simulink model "vehicleXYsim"  (R2018b)
settings: Solver=FixedStepAuto  StartTime=0.0  StopTime=end_time  FixedStep=0.1  RelTol=1e-3
libraries: simulink x2, vehdynlibviscommon x1
settings Model: Creator=mk  LastModifiedBy=mk

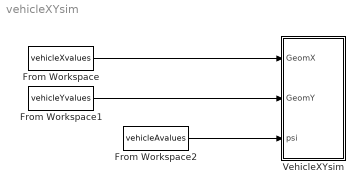
== system vehicleXYsim ==
  From Workspace : FromWorkspace  VariableName=vehicleXvalues  SampleTime=0
  From Workspace1 : FromWorkspace  VariableName=vehicleYvalues  SampleTime=0
  From Workspace2 : FromWorkspace  VariableName=vehicleAvalues  SampleTime=0
  VehicleXYsim : Subsystem
  wires:
  From Workspace/1 -> VehicleXYsim/1(GeomX)
  From Workspace1/1 -> VehicleXYsim/2(GeomY)
  From Workspace2/1 -> VehicleXYsim/3(psi)

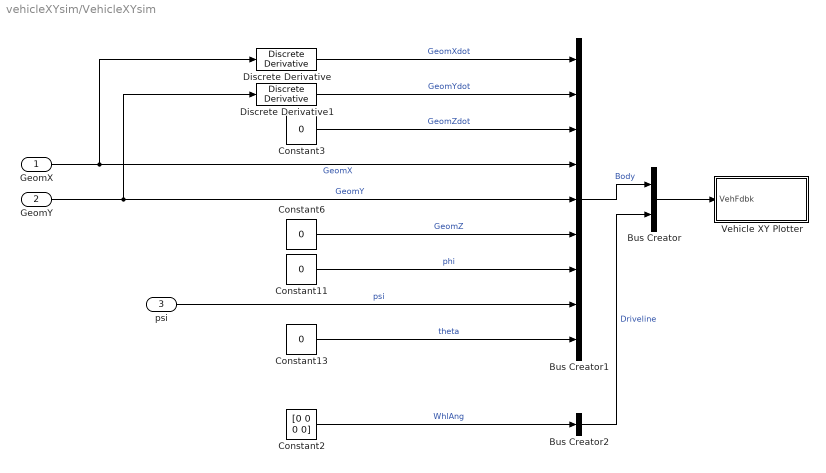
== system vehicleXYsim/VehicleXYsim ==
  GeomX : Inport
  GeomY : Inport  Port=2
  psi : Inport  Port=3
  Bus Creator : BusCreator  Inputs=2
  Bus Creator1 : BusCreator  Inputs=9
  Bus Creator2 : BusCreator  Inputs=1
  Constant{3,6,11,13} (4 alike) : Constant  Value=0
  Constant2 : Constant  Value=[0 0 0 0]
  Discrete Derivative : simulink/Discrete/Discrete Derivative  gainval=1.0  ICPrevScaledInput=0.0  OutMin=[]  OutMax=[]  OutDataType=fixdt(1, 16)  OutScaling=2^-10  DoSatur=off
  Discrete Derivative1 : simulink/Discrete/Discrete Derivative  gainval=1.0  ICPrevScaledInput=0.0  OutMin=[]  OutMax=[]  OutDataType=fixdt(1, 16)  OutScaling=2^-10  DoSatur=off
  Vehicle XY Plotter : Subsystem  mask(Vehicle XY Plotter){a=0.5, b=0.5, w=0.75, figBorder=10, bufferSize=1024, pltDT=.1}
      mask prompts: a "Distance to front axle from CG, a [m]:"; b "Distance to rear axle from CG, b [m]:"; w "Track width, w [m]:"; figBorder "Distance to figure borders, figBorder [m]:"; bufferSize "Path buffer sampe size, bufferSize []:"; pltDT "Plot update rate, pltDT [s]:"
      mask help: This block will display a MATLAB figure which indicates the vehicle path, current position and heading velocity.
      mask TypeOptions a: Vehicle XY Plotter/a
      mask TypeOptions b: Vehicle XY Plotter/b
      mask TypeOptions w: Vehicle XY Plotter/w
      mask TypeOptions figBorder: Vehicle XY Plotter/figBorder
      mask TypeOptions bufferSize: Vehicle XY Plotter/bufferSize
  wires:
  Discrete Derivative/1 -> Bus Creator1/1  "GeomXdot"
  GeomY/1 -> Discrete Derivative1/1, Bus Creator1/5  "GeomY"
  Constant3/1 -> Bus Creator1/3  "GeomZdot"
  Constant6/1 -> Bus Creator1/6  "GeomZ"
  GeomX/1 -> Discrete Derivative/1, Bus Creator1/4  "GeomX"
  Constant11/1 -> Bus Creator1/7  "phi"
  Constant2/1 -> Bus Creator2/1  "WhlAng"
  Constant13/1 -> Bus Creator1/9  "theta"
  Discrete Derivative1/1 -> Bus Creator1/2  "GeomYdot"
  Bus Creator2/1 -> Bus Creator/2  "Driveline"
  Bus Creator/1 -> Vehicle XY Plotter/1(VehFdbk)
  psi/1 -> Bus Creator1/8  "psi"
  Bus Creator1/1 -> Bus Creator/1  "Body"

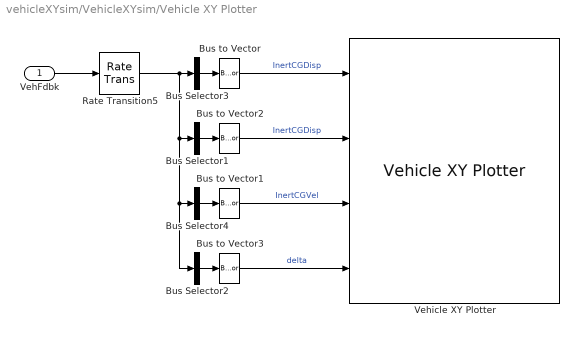
== system vehicleXYsim/VehicleXYsim/Vehicle XY Plotter ==
  VehFdbk : Inport
  Bus Selector1 : BusSelector  OutputSignals=Body.phi,Body.theta,Body.psi  OutputAsBus=on
  Bus Selector2 : BusSelector  OutputSignals=Driveline.WhlAng  OutputAsBus=on
  Bus Selector3 : BusSelector  OutputSignals=Body.GeomX,Body.GeomY,Body.GeomZ  OutputAsBus=on
  Bus Selector4 : BusSelector  OutputSignals=Body.GeomXdot,Body.GeomYdot,Body.GeomZdot  OutputAsBus=on
  Bus to Vector{,1..3} (4 alike) : BusToVector
  Rate Transition5 : RateTransition  Deterministic=off  OutPortSampleTime=pltDT
  Vehicle XY Plotter : vehdynlibviscommon/Vehicle XY Plotter  bufferSize=bufferSize  w=w  a=a  b=b  figBorder=figBorder
  wires:
  Bus to Vector2/1 -> Vehicle XY Plotter/2  "InertCGDisp"
  Bus Selector4/1 -> Bus to Vector1/1
  Bus to Vector1/1 -> Vehicle XY Plotter/3  "InertCGVel"
  Bus Selector1/1 -> Bus to Vector2/1
  Bus to Vector/1 -> Vehicle XY Plotter/1  "InertCGDisp"
  Bus Selector3/1 -> Bus to Vector/1
  Bus Selector2/1 -> Bus to Vector3/1
  VehFdbk/1 -> Rate Transition5/1
  Bus to Vector3/1 -> Vehicle XY Plotter/4  "delta"
  Rate Transition5/1 -> Bus Selector1/1, Bus Selector2/1, Bus Selector4/1, Bus Selector3/1
